simulink model "BatteryModelDifferentialEquationsWithSoE"  (R2023b)
settings: Solver=VariableStepAuto  StartTime=0.0  StopTime=3600  RelTol=1e-3
values from neighbouring files (symbols this model uses):
  C1 = 12.6138    [DPBatteryDynamics.m]    (also in DPBatteryModuleDynamics.m = 174.354594213; MPCControllerForModuleSim.m = 174.354594213; StateSpaceScript.m; TubeBasedMPCControllerForModuleSim.m = 174.354594213)
  Cc = 62.7    [DPBatteryDynamics.m]    (also in DPBatteryModuleDynamics.m = 2059.88437317; MPCControllerForModuleSim.m = 2059.88437317; StateSpaceScript.m; TubeBasedMPCControllerForModuleSim.m = 2059.88437317)
  Cn = 78    [DPBatteryDynamics.m]    (also in DPBatteryModuleDynamics.m = 156; MPCControllerForModuleSim.m = 156; StateSpaceScript.m; TubeBasedMPCControllerForModuleSim.m = 156)
  Cs = 4.5    [DPBatteryDynamics.m]    (also in DPBatteryModuleDynamics.m = 31.8813725212; MPCControllerForModuleSim.m = 31.8813725212; StateSpaceScript.m; TubeBasedMPCControllerForModuleSim.m = 31.8813725212)
  ENom = 1056908.83315503    (= 1056908.83316)    [DPBatteryDynamics.m]    (also in DPBatteryModuleDynamics.m = 24521235.1894; FMINCONControllerForCellSim.m = 992623.375585; MPCControllerForModuleSim.m = 24521235.1894; TubeBasedMPCControllerForCellSim.m = 992623.375585)
  IBar = sqrt(Cc*(TcBar - TsBar) / (Rc*Cc*(R1+R0)))    [StateSpaceScript.m]
  R0 = 0.0099131    [DPBatteryDynamics.m]    (also in DPBatteryModuleDynamics.m = 0.000127631043389; FMINCONControllerForCellSim.m = 0.00292724690916; MPCControllerForModuleSim.m = 0.000127631043389; StateSpaceScript.m)
  R1 = 3e-4    (= 0.0003)    [DPBatteryDynamics.m]    (also in DPBatteryModuleDynamics.m = 0.00360795873337; MPCControllerForModuleSim.m = 0.00360795873337; StateSpaceScript.m; TubeBasedMPCControllerForModuleSim.m = 0.00360795873337)
  Rc = 1.94    [DPBatteryDynamics.m]    (also in DPBatteryModuleDynamics.m = 14.480191951; MPCControllerForModuleSim.m = 14.480191951; StateSpaceScript.m; TubeBasedMPCControllerForModuleSim.m = 14.480191951)
  Ru = 15    [DPBatteryDynamics.m]    (also in DPBatteryModuleDynamics.m = 8.86466905699; MPCControllerForModuleSim.m = 8.86466905699; StateSpaceScript.m; TubeBasedMPCControllerForModuleSim.m = 8.86466905699)
  soc_ocv_coefficients = [-2.0713 4.5787 -2.7974 0.9751 3.4939]'    [DPBatteryDynamics.m]    (also in DPBatteryModuleDynamics.m; FMINCONControllerForCellSim.m; MPCControllerForModuleSim.m = [-24.9533 55.1604 -33.8647 11.9152 41.5814]'; TubeBasedMPCControllerForCellSim.m)
  Tf = 20    [DPBatteryDynamics.m]    (also in DPBatteryModuleDynamics.m; MPCControllerForModuleSim.m; RHC_test.m; StateSpaceScript.m)
undefined symbols (not defined in the file or in its folder): sim_time
libraries: simulink x1
settings Model: Creator=adamb  LastModifiedBy=Adam

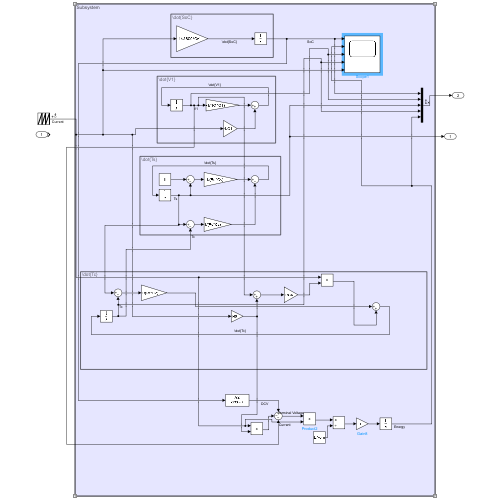
[thumbnail: Simulink's stored preview of the top-level diagram]
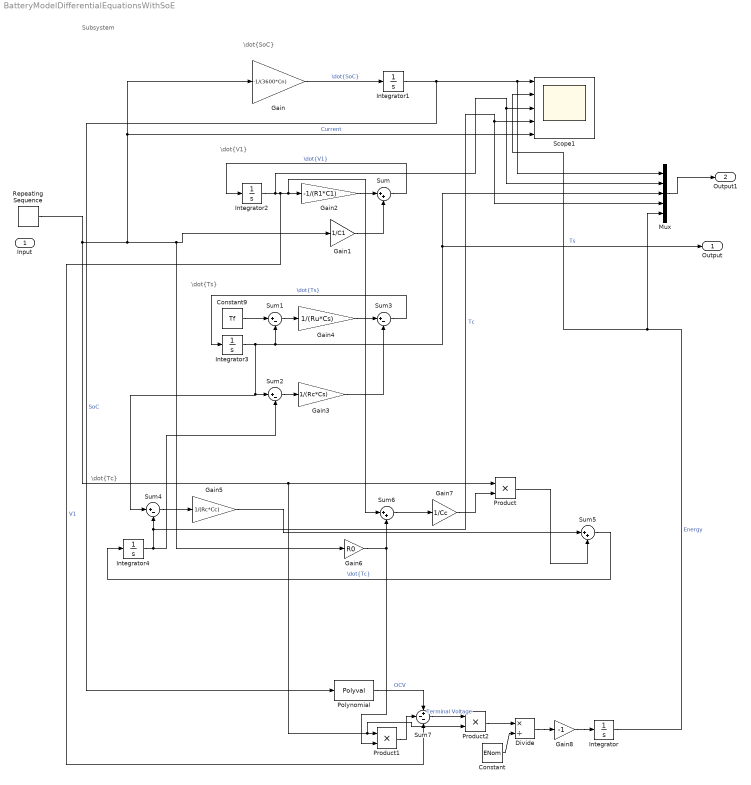
== system BatteryModelDifferentialEquationsWithSoE ==
  note: Subsystem
  note: \dot{V1}
  note: \dot{SoC}
  note: \dot{Ts}
  note: \dot{Tc}
  Input : Inport
  Constant : Constant  Value=ENom
  Constant9 : Constant  Value=Tf
  Divide : Product  Inputs=*/
  Gain : Gain  Gain=-1/(3600*Cn)
  Gain1 : Gain  Gain=1/C1
  Gain2 : Gain  Gain=-1/(R1*C1)
  Gain3 : Gain  Gain=1/(Rc*Cs)
  Gain4 : Gain  Gain=1/(Ru*Cs)
  Gain5 : Gain  Gain=1/(Rc*Cc)
  Gain6 : Gain  Gain=R0
  Gain7 : Gain  Gain=1/Cc
  Gain8 : Gain  Gain=-1
  Integrator : Integrator  InitialCondition=1
  Integrator1 : Integrator  InitialCondition=1
  Integrator2 : Integrator
  Integrator3 : Integrator  InitialCondition=Tf
  Integrator4 : Integrator  InitialCondition=Tf
  Mux : Mux  Inputs=5
  Polynomial : Polyval  Coefs=soc_ocv_coefficients
  Product : Product
  Product1 : Product
  Product2 : Product
  Repeating Sequence : simulink/Sources/Repeating Sequence  rep_seq_t=sim_time  rep_seq_y=IBar*ones(size(sim_time))
  Scope1 : Scope  NumInputPorts=5
  Sum : Sum  Inputs=|++
  Sum{1..4} (4 alike) : Sum  Inputs=|+-
  Sum5 : Sum  Inputs=|++
  Sum6 : Sum  Inputs=|++
  Sum7 : Sum  Inputs=+--
  Output : Outport  PortDimensions=2
  Output1 : Outport  Port=2
  wires:
  Sum3/1 -> Integrator3/1  "\\dot{Ts}"
  Sum2/1 -> Gain3/1
  Sum1/1 -> Gain4/1
  Product/1 -> Sum5/2
  Gain/1 -> Integrator1/1  "\\dot{SoC}"
  Gain2/1 -> Sum/1
  Gain7/1 -> Product/2
  Gain5/1 -> Sum5/1
  Constant9/1 -> Sum1/1
  Integrator2/1 -> Sum7/3, Sum6/1, Gain2/1, Scope1/3, Mux/2  "V1"
  Gain6/1 -> Product1/2, Sum6/2
  Gain3/1 -> Sum3/2
  Sum4/1 -> Gain5/1
  Integrator3/1 -> Sum4/1, Sum2/1, Mux/3, Output/1, Sum1/2  "Ts"
  Sum5/1 -> Integrator4/1  "\\dot{Tc}"
  Integrator1/1 -> Polynomial/1, Mux/1, Scope1/1  "SoC"
  Integrator4/1 -> Sum2/2, Scope1/4, Mux/4, Sum4/2  "Tc"
  Sum/1 -> Integrator2/1  "\\dot{V1}"
  Sum6/1 -> Gain7/1
  Gain4/1 -> Sum3/1
  Gain1/1 -> Sum/2
  Mux/1 -> Output1/1
  Repeating Sequence/1 -> Product2/2, Product1/1, Product/1, Gain1/1, Gain6/1, Gain/1, Scope1/5  "Current"
  Polynomial/1 -> Sum7/1  "OCV"
  Product1/1 -> Sum7/2
  Sum7/1 -> Product2/1  "Terminal Voltage"
  Product2/1 -> Divide/1
  Integrator/1 -> Mux/5, Scope1/2  "Energy"
  Gain8/1 -> Integrator/1
  Constant/1 -> Divide/2
  Divide/1 -> Gain8/1
